simulink model "PWM_Rectifier_3phase_sensless"  (R2019b)
settings: Solver=ode45  StartTime=0.0  StopTime=2  MaxStep=2e-6  RelTol=1e-3  EnableMultiTasking=on
InitFcn:
  | clear;
  | clc;
  | f=50;
  | Vp=220*sqrt(2);
  | fs=20e3;
  | k=0.1;
libraries: powerlib x25, powerlib_meascontrol x10, simulink x3
settings Model: Creator=Syed Abdul Rahman  LastModifiedBy=Stan
settings DataIOCC: LimitDataPoints=on  SaveFormat=Array  ReturnWorkspaceOutputs=off
settings OptimizationCC: ExpressionDepthLimit=2147483647  LifeSpan=inf
settings DebuggingCC: UnderspecifiedInitializationDetection=Classic  MergeDetectMultiDrivingBlocksExec=none  SolverPrmCheckMsg=warning  FcnCallInpInsideContextMsg=warning  StateNameClashWarn=warning  SFUnexpectedBacktrackingDiag=warning  SFNoUnconditionalDefaultTransitionDiag=warning  SFExecutionAtInitializationDiag=none  ArithmeticOperatorsInVariantConditions=warning
settings HardwareCC: ProdBitPerPointer=32  ProdBitPerSizeT=32  ProdBitPerPtrDiffT=32  ProdLargestAtomicFloat=None  ProdIntDivRoundTo=Undefined  ProdEndianess=Unspecified  ProdWordSize=32  ProdHWDeviceType=32-bit Generic
settings ModelReferenceCC: PropagateSignalLabelsOutOfModel=off
settings SFSimCC: SimUseLocalCustomCode=off  CustomCodeUndefinedFunction=UseInterfaceOnly
settings RTWCC: RTWUseLocalCustomCode=off
settings CodeAppCC: StateflowObjectComments=on
settings GRTTargetCC: TargetLangStandard=C89/C90 (ANSI)  GeneratePreprocessorConditionals=Disable all  CombineOutputUpdateFcns=off  GRTInterface=on
settings ConfigComp: CovMetricSettings=dw  CovHtmlReporting=on  CovSaveCumulativeToWorkspaceVar=on  CovSaveSingleToWorkspaceVar=on  CovExternalEMLEnable=off
settings SimscapeCC: SimscapeLogType=all  SimscapeLogToSDI=on

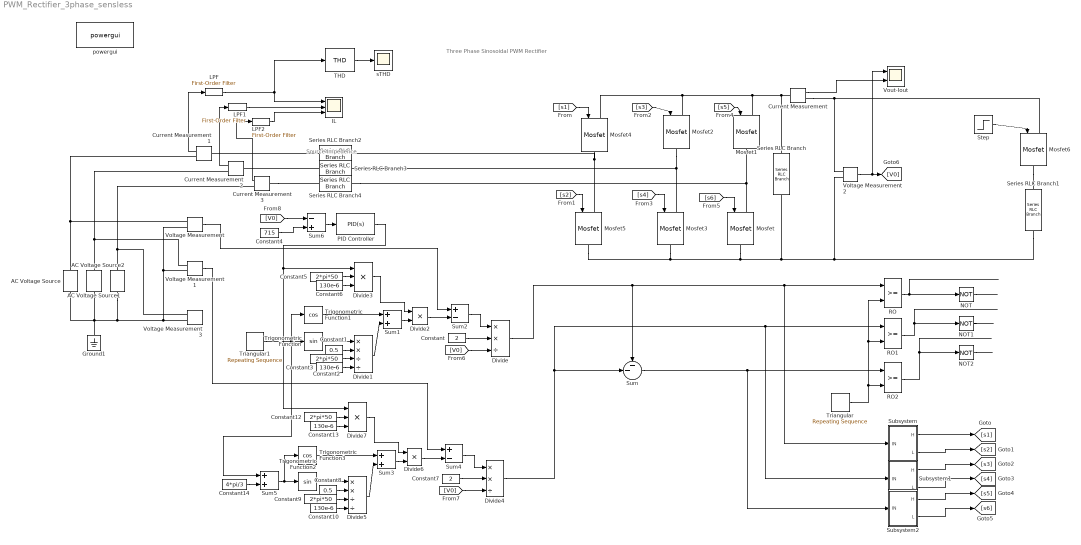
== system PWM_Rectifier_3phase_sensless ==
  note: Three Phase Sinosoidal PWM Rectifier
  note: Source Impedence
  AC Voltage Source : powerlib/Electrical Sources/AC Voltage Source  Amplitude=Vp  Phase=0  Frequency=f  SampleTime=0  Measurements=None  BusType=swing  Pref=10e3  Qref=0  Qmin=-inf  Qmax=+inf
      settings: SourceProductName=Simscape Electrical
  AC Voltage Source1 : powerlib/Electrical Sources/AC Voltage Source  Amplitude=Vp  Phase=240  Frequency=f  SampleTime=0  Measurements=None  BusType=swing  Pref=10e3  Qref=0  Qmin=-inf  Qmax=+inf
      settings: SourceProductName=Simscape Electrical
  AC Voltage Source2 : powerlib/Electrical Sources/AC Voltage Source  Amplitude=Vp  Phase=120  Frequency=f  SampleTime=0  Measurements=None  BusType=swing  Pref=10e3  Qref=0  Qmin=-inf  Qmax=+inf
      settings: SourceProductName=Simscape Electrical
  Constant : Constant  Value=2
  Constant1 : Constant  Value=0.5
  Constant{3,6,10,13} (4 alike) : Constant  Value=130e-6
  Constant{2,5,9,12} (4 alike) : Constant  Value=2*pi*50
  Constant14 : Constant  Value=4*pi/3
  Constant4 : Constant  Value=715
  Constant7 : Constant  Value=2
  Constant8 : Constant  Value=0.5
  Current Measurement{,1..3} (4 alike) : powerlib/Measurements/Current Measurement  PhasorSimulation=off  OutputType=Complex  PSBequivalent=0
      settings: SourceProductName=Simscape Electrical
  Divide : Product  Inputs=**/
  Divide1 : Product  Inputs=**//
  Divide2 : Product  Inputs=**
  Divide3 : Product  Inputs=***
  Divide4 : Product  Inputs=**/
  Divide5 : Product  Inputs=**//
  Divide6 : Product  Inputs=**
  Divide7 : Product  Inputs=***
  Ground1 : powerlib/Elements/Ground  LConnTagsString=a
      settings: SourceProductName=Simscape Electrical
  "IL " : Scope  NumInputPorts=3
  LPF : powerlib_meascontrol/Filters/First-Order Filter  FilterType=Lowpass  Tc=1/(2*pi*0.5e3)  Ts=0  Initialize=off  Vac_Init=[0, 0, 60]  Vdc_Init=0  PlotResponse=off  FreqRange="[0,  200,  1]"
      settings: SourceProductName=Simscape Electrical
  LPF1 : powerlib_meascontrol/Filters/First-Order Filter  FilterType=Lowpass  Tc=1/(2*pi*0.5e3)  Ts=0  Initialize=off  Vac_Init=[0, 0, 60]  Vdc_Init=0  PlotResponse=off  FreqRange="[0,  200,  1]"
      settings: SourceProductName=Simscape Electrical
  LPF2 : powerlib_meascontrol/Filters/First-Order Filter  FilterType=Lowpass  Tc=1/(2*pi*0.5e3)  Ts=0  Initialize=off  Vac_Init=[0, 0, 60]  Vdc_Init=0  PlotResponse=off  FreqRange="[0,  200,  1]"
      settings: SourceProductName=Simscape Electrical
  Mosfet{,1..6} (7 alike) : powerlib/Power Electronics/Mosfet  Ron=0.1  Lon=0  Rd=0.01  Vfd=0  IC=0  Rs=1e5  Cs=inf  Measurements=off
      settings: SourceProductName=Simscape Electrical
  NOT : Logic  Operator=NOT  IconShape=distinctive  AllPortsSameDT=off  OutDataTypeStr=boolean
  NOT1 : Logic  Operator=NOT  IconShape=distinctive  AllPortsSameDT=off  OutDataTypeStr=boolean
  NOT2 : Logic  Operator=NOT  IconShape=distinctive  AllPortsSameDT=off  OutDataTypeStr=boolean
  PID Controller : simulink/Continuous/PID Controller  Controller=PID  Form=Parallel  TimeDomain=Continuous-time  SampleTime=-1  IntegratorMethod=Forward Euler  FilterMethod=Forward Euler  ControllerParametersSource=internal  P=10  I=100  D=0  UseFilter=on  N=100  TunerSelectOption=Transfer Function Based (PID Tuner App)  InitialConditionSource=internal  InitialConditionForIntegrator=0  InitialConditionForFilter=0  DifferentiatorICPrevScaledInput=0  ExternalReset=none  TrackingMode=off  Kt=1  LimitOutput=on  UpperSaturationLimit=300  LowerSaturationLimit=-300  LinearizeAsGain=on  AntiWindupMode=none  Kb=1  POutMin=[]  POutMax=[]  IOutMin=[]  IOutMax=[]  DOutMin=[]  DOutMax=[]  NOutMin=[]  NOutMax=[]  SumOutMin=[]  SumOutMax=[]  SaturationOutMin=[]  SaturationOutMax=[]  PParamMin=[]  PParamMax=[]  IParamMin=[]  IParamMax=[]  DParamMin=[]  DParamMax=[]  NParamMin=[]  NParamMax=[]  KbParamMin=[]  KbParamMax=[]  KtParamMin=[]  KtParamMax=[]  KbOutMin=[]  KbOutMax=[]  KtOutMin=[]  KtOutMax=[]  IntegratorOutMin=[]  IntegratorOutMax=[]  FilterOutMin=[]  FilterOutMax=[]  SumI1OutMin=[]  SumI1OutMax=[]  SumI2OutMin=[]  SumI2OutMax=[]  SumI3OutMin=[]  SumI3OutMax=[]  SumI4OutMin=[]  SumI4OutMax=[]  SumDOutMin=[]  SumDOutMax=[]  DifferentiatorOutMin=[]  DifferentiatorOutMax=[]  FilterDiffOutCoefMin=[]  FilterDiffOutCoefMax=[]  ReciprocalOutMin=[]  ReciprocalOutMax=[]  SumDenOutMin=[]  SumDenOutMax=[]  SumNumOutMin=[]  SumNumOutMax=[]  DivideOutMin=[]  DivideOutMax=[]  IntegratorContinuousStateAttributes=''  IntegratorStateMustResolveToSignalObject=off  IntegratorRTWStateStorageClass=Auto  FilterContinuousStateAttributes=''  FilterStateMustResolveToSignalObject=off  FilterRTWStateStorageClass=Auto  ParallelPVariant=InternalParameters  IdealPVariant=Disabled  IVariant=InternalParameters  DVariant=InternalParameters  IntegratorVariant=Continuous  SatVariant=Enabled  AWVariant=Passthrough  PCopyVariant=Disabled  TRVariant=Disabled  FdbkBlocksVariant=Forward  IdealPFdbkVariant=Disabled  SatFdbkVariant=Disabled  DerivativeFilterVariant=ContFilter  NVariant=InternalParameters  NCopyVariant=Disabled  FilterICVariant=InternalICsFilter  IntegratorICVariant=InternalICs  ExternalResetVariant=Disabled  TRSumVariant=Passthrough  SumFdbkVariant=Disabled  SumVariant=Sum_PID
  RO : RelationalOperator  OutDataTypeStr=boolean  RndMeth=Nearest
  RO1 : RelationalOperator  OutDataTypeStr=boolean  RndMeth=Nearest
  RO2 : RelationalOperator  OutDataTypeStr=boolean  RndMeth=Nearest
  Series RLC Branch : powerlib/Elements/Series RLC Branch  LConnTagsString=__new0  RConnTagsString=__new0  BranchType=C  Resistance=5  Inductance=1e-3  SetiL0=off  InitialCurrent=0  Capacitance=470e-3  Setx0=on  InitialVoltage=700  Measurements=None
      settings: SourceProductName=Simscape Electrical
  Series RLC Branch1 : powerlib/Elements/Series RLC Branch  LConnTagsString=__new0  RConnTagsString=__new0  BranchType=R  Resistance=20  Inductance=1e-3  SetiL0=off  InitialCurrent=0  Capacitance=200e-6  Setx0=off  InitialVoltage=0  Measurements=None
      settings: SourceProductName=Simscape Electrical
  Series RLC Branch2 : powerlib/Elements/Series RLC Branch  LConnTagsString=__new0  RConnTagsString=__new0  BranchType=RL  Resistance=0.5  Inductance=130e-6  SetiL0=off  InitialCurrent=0  Capacitance=200e-6  Setx0=off  InitialVoltage=0  Measurements=None
      settings: SourceProductName=Simscape Electrical
  Series RLC Branch3 : powerlib/Elements/Series RLC Branch  LConnTagsString=__new0  RConnTagsString=__new0  BranchType=RL  Resistance=0.5  Inductance=130e-6  SetiL0=off  InitialCurrent=0  Capacitance=200e-6  Setx0=off  InitialVoltage=0  Measurements=None
      settings: SourceProductName=Simscape Electrical
  Series RLC Branch4 : powerlib/Elements/Series RLC Branch  LConnTagsString=__new0  RConnTagsString=__new0  BranchType=RL  Resistance=0.5  Inductance=130e-6  SetiL0=off  InitialCurrent=0  Capacitance=200e-6  Setx0=off  InitialVoltage=0  Measurements=None
      settings: SourceProductName=Simscape Electrical
  Step : Step  SampleTime=0
  Subsystem : Subsystem
  Subsystem1 : Subsystem
  Subsystem2 : Subsystem
  Sum : Sum  Inputs=--|
  Sum1 : Sum
  Sum2 : Sum  Inputs=+-
  Sum3 : Sum
  Sum4 : Sum  Inputs=+-
  Sum5 : Sum
  Sum6 : Sum  Inputs=-+
  THD : powerlib_meascontrol/Measurements/THD  Freq=50  Ts=0
      settings: SourceProductName=Simscape Electrical
  Triangular : simulink/Sources/Repeating Sequence  rep_seq_t="[0  1/(10e3)]"  rep_seq_y=[-1 1]
  Triangular1 : simulink/Sources/Repeating Sequence  rep_seq_t="[0  1/(50)]"  rep_seq_y=[0 2*pi]
  Trigonometric Function : Trigonometry
  Trigonometric Function1 : Trigonometry  Operator=cos
  Trigonometric Function2 : Trigonometry
  Trigonometric Function3 : Trigonometry  Operator=cos
  Voltage Measurement{,1..3} (4 alike) : powerlib/Measurements/Voltage Measurement  PhasorSimulation=off  OutputType=Complex  PSBequivalent=0
      settings: SourceProductName=Simscape Electrical
  Vout-Iout : Scope  NumInputPorts=2
  powergui : powerlib/powergui  Priority=1  SimulationMode=Discrete  SampleTime=2e-6  frequency=60  Iterations=50  frequencyindice=50  Pbase=100e6  ErrMax=1e-4  UnitsV=kV  UnitsW=MW  buscounter=0  FunctionMessages=off  echomessages=off  EnableUseOfTLC=off  CurrentSourceSwitches=off  DisableSnubberDevices=off  DisableRonSwitches=off  DisableVfSwitches=off  DisplayEquations=off  AutomaticDiscreteSolvers=off  SolverType=Tustin/Backward Euler (TBE)  Interpol=off  ExternalGateDelay=off  methode=off  Ts=0  x0status=blocks  SPID=off  SwTol=0  HookPort=off  NonlinearTolerance=1e-4  nMaxIteration=100  ContinueOnMaxIteration=off  RestoreLinks=warning  ResistiveCurrentMeasurement=off  Frange=[0:2:500]  Ylog=off  Xlog=on  ShowGrid=off  save=off  variable=ZData  structure=0  ZoomFFT=on  StartTime=0.0  cycles=1  DisplayStyle=1  fundamental=60  FreqAxis=off  MaxFrequency=1000  frequencyindicesteady=1  RmsSteady=1  display=off
      settings: SourceProductName=Simscape Electrical
  sTHD : Scope
  wires:
  [s1] -> Mosfet4/1
  [s2] -> Mosfet5/1
  [s3] -> Mosfet2/1
  [s4] -> Mosfet3/1
  [s5] -> Mosfet1/1
  [s6] -> Mosfet/1
  Voltage Measurement/1 -> Sum2/1
  Voltage Measurement2/1 -> Vout-Iout/1, [V0]
  NOT/1 -> ?
  NOT1/1 -> ?
  NOT2/1 -> ?
  RO/1 -> NOT/1
  RO1/1 -> NOT1/1
  Sum/1 -> Subsystem2/1(IN), RO2/1
  RO2/1 -> NOT2/1
  Current Measurement1/1 -> LPF/1
  LPF/1 -> THD/1, "IL "/1
  LPF1/1 -> "IL "/2
  Current Measurement2/1 -> LPF1/1
  LPF2/1 -> "IL "/3
  Current Measurement3/1 -> LPF2/1
  [V0] -> Divide/3
  Constant/1 -> Divide/2
  Divide/1 -> Sum/1, Subsystem/1(IN), RO/1
  Trigonometric Function/1 -> Divide1/1
  Constant1/1 -> Divide1/2
  Constant2/1 -> Divide1/3
  Constant3/1 -> Divide1/4
  Divide1/1 -> Sum1/2
  Trigonometric Function1/1 -> Sum1/1
  Sum1/1 -> Divide2/2
  Divide3/1 -> Divide2/1
  Constant6/1 -> Divide3/3
  Constant5/1 -> Divide3/2
  Divide2/1 -> Sum2/2
  Sum2/1 -> Divide/1
  Sum4/1 -> Divide4/1
  Divide6/1 -> Sum4/2
  PID Controller/1 -> Divide3/1, Divide7/1
  Constant12/1 -> Divide7/2
  Constant13/1 -> Divide7/3
  Divide7/1 -> Divide6/1
  Sum3/1 -> Divide6/2
  Trigonometric Function3/1 -> Sum3/1
  Divide5/1 -> Sum3/2
  Constant10/1 -> Divide5/4
  Constant9/1 -> Divide5/3
  Constant8/1 -> Divide5/2
  Trigonometric Function2/1 -> Divide5/1
  Constant7/1 -> Divide4/2
  [V0] -> Divide4/3
  Voltage Measurement1/1 -> Sum4/1
  Sum5/1 -> Trigonometric Function3/1, Trigonometric Function2/1
  Constant14/1 -> Sum5/2
  Triangular1/1 -> Sum5/1, Trigonometric Function1/1, Trigonometric Function/1
  Divide4/1 -> Subsystem1/1(IN), RO1/1, Sum/2
  Triangular/1 -> RO1/2, RO/2, RO2/2
  Sum6/1 -> PID Controller/1
  Constant4/1 -> Sum6/2
  [V0] -> Sum6/1
  Step/1 -> Mosfet6/1
  Subsystem/1(H) -> [s1]
  Subsystem/2(L) -> [s2]
  Subsystem1/1(H) -> [s3]
  Subsystem1/2(L) -> [s4]
  Subsystem2/1(H) -> [s5]
  Subsystem2/2(L) -> [s6]
  THD/1 -> sTHD/1
  Current Measurement/1 -> Vout-Iout/2
  connections:
  Series RLC Branch/LConn1 -- Mosfet1/LConn1 -- Mosfet2/LConn1 -- Mosfet4/LConn1 -- Current Measurement/LConn1
  Mosfet4/RConn1 -- Mosfet5/LConn1 -- Series RLC Branch2/LConn1
  Mosfet/LConn1 -- Series RLC Branch4/LConn1 -- Mosfet1/RConn1
  Series RLC Branch1/RConn1 -- Voltage Measurement2/LConn2 -- Mosfet3/RConn1 -- Mosfet5/RConn1 -- Mosfet/RConn1 -- Series RLC Branch/RConn1
  Mosfet2/RConn1 -- Mosfet3/LConn1 -- Series RLC Branch3/LConn1
  AC Voltage Source/LConn1 -- AC Voltage Source2/LConn1 -- Voltage Measurement1/LConn2 -- Voltage Measurement/LConn2 -- Voltage Measurement3/LConn2 -- AC Voltage Source1/LConn1 -- Ground1/LConn1
  Current Measurement1/RConn1 -- Voltage Measurement/LConn1 -- AC Voltage Source/RConn1
  Voltage Measurement1/LConn1 -- Current Measurement2/RConn1 -- AC Voltage Source1/RConn1
  Current Measurement3/RConn1 -- Voltage Measurement3/LConn1 -- AC Voltage Source2/RConn1
  Current Measurement/RConn1 -- Mosfet6/LConn1 -- Voltage Measurement2/LConn1
  Current Measurement1/LConn1 -- Series RLC Branch2/RConn1
  Current Measurement3/LConn1 -- Series RLC Branch4/RConn1
  Series RLC Branch3/RConn1 -- Current Measurement2/LConn1
  Mosfet6/RConn1 -- Series RLC Branch1/LConn1

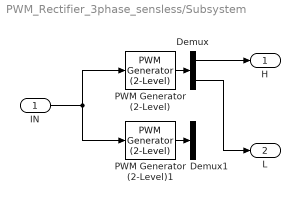
== system PWM_Rectifier_3phase_sensless/Subsystem ==
  IN : Inport
  Demux : Demux  Outputs=2
  Demux1 : Demux  Outputs=2
  PWM Generator (2-Level) : powerlib_meascontrol/Pulse & Signal Generators/PWM Generator (2-Level)  ModulatorType=Single-phase half-bridge (2 pulses)  ModulatorMode=Unsynchronized  Fc=20000  Pc=90  nF=27  MinMax="[-1  1]"  SamplingTechnique=Natural  ModulatingSignals=off  m=0.8  Freq=60  Phase=0  Ts=0  ShowCarrierOutport=off
  PWM Generator (2-Level)1 : powerlib_meascontrol/Pulse & Signal Generators/PWM Generator (2-Level)  ModulatorType=Single-phase half-bridge (2 pulses)  ModulatorMode=Unsynchronized  Fc=20000  Pc=90  nF=27  MinMax=[-1 -1e-4]  SamplingTechnique=Natural  ModulatingSignals=off  m=0.8  Freq=60  Phase=0  Ts=0  ShowCarrierOutport=off
  H : Outport  VectorParamsAs1DForOutWhenUnconnected=off
  L : Outport  Port=2  VectorParamsAs1DForOutWhenUnconnected=off
  wires:
  Demux/1 -> H/1
  IN/1 -> PWM Generator (2-Level)1/1, PWM Generator (2-Level)/1
  PWM Generator (2-Level)1/1 -> Demux1/1
  PWM Generator (2-Level)/1 -> Demux/1
  Demux/2 -> L/1

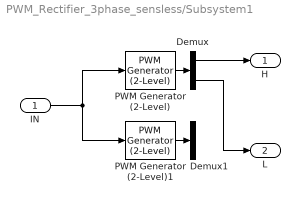
== system PWM_Rectifier_3phase_sensless/Subsystem1 ==
  IN : Inport
  Demux : Demux  Outputs=2
  Demux1 : Demux  Outputs=2
  PWM Generator (2-Level) : powerlib_meascontrol/Pulse & Signal Generators/PWM Generator (2-Level)  ModulatorType=Single-phase half-bridge (2 pulses)  ModulatorMode=Unsynchronized  Fc=20000  Pc=90  nF=27  MinMax="[-1  1]"  SamplingTechnique=Natural  ModulatingSignals=off  m=0.8  Freq=60  Phase=0  Ts=0  ShowCarrierOutport=off
  PWM Generator (2-Level)1 : powerlib_meascontrol/Pulse & Signal Generators/PWM Generator (2-Level)  ModulatorType=Single-phase half-bridge (2 pulses)  ModulatorMode=Unsynchronized  Fc=20000  Pc=90  nF=27  MinMax=[-1 -1e-4]  SamplingTechnique=Natural  ModulatingSignals=off  m=0.8  Freq=60  Phase=0  Ts=0  ShowCarrierOutport=off
  H : Outport  VectorParamsAs1DForOutWhenUnconnected=off
  L : Outport  Port=2  VectorParamsAs1DForOutWhenUnconnected=off
  wires:
  Demux/2 -> L/1
  PWM Generator (2-Level)/1 -> Demux/1
  PWM Generator (2-Level)1/1 -> Demux1/1
  IN/1 -> PWM Generator (2-Level)/1, PWM Generator (2-Level)1/1
  Demux/1 -> H/1

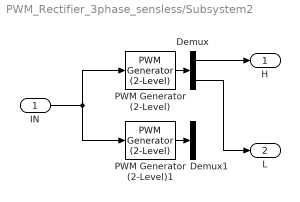
== system PWM_Rectifier_3phase_sensless/Subsystem2 ==
  IN : Inport
  Demux : Demux  Outputs=2
  Demux1 : Demux  Outputs=2
  PWM Generator (2-Level) : powerlib_meascontrol/Pulse & Signal Generators/PWM Generator (2-Level)  ModulatorType=Single-phase half-bridge (2 pulses)  ModulatorMode=Unsynchronized  Fc=20000  Pc=90  nF=27  MinMax="[-1  1]"  SamplingTechnique=Natural  ModulatingSignals=off  m=0.8  Freq=60  Phase=0  Ts=0  ShowCarrierOutport=off
  PWM Generator (2-Level)1 : powerlib_meascontrol/Pulse & Signal Generators/PWM Generator (2-Level)  ModulatorType=Single-phase half-bridge (2 pulses)  ModulatorMode=Unsynchronized  Fc=20000  Pc=90  nF=27  MinMax=[-1 -1e-4]  SamplingTechnique=Natural  ModulatingSignals=off  m=0.8  Freq=60  Phase=0  Ts=0  ShowCarrierOutport=off
  H : Outport  VectorParamsAs1DForOutWhenUnconnected=off
  L : Outport  Port=2  VectorParamsAs1DForOutWhenUnconnected=off
  wires:
  Demux/1 -> H/1
  IN/1 -> PWM Generator (2-Level)1/1, PWM Generator (2-Level)/1
  PWM Generator (2-Level)1/1 -> Demux1/1
  PWM Generator (2-Level)/1 -> Demux/1
  Demux/2 -> L/1
